simulink model "EKF_MODEL_needfix"  (R2023b)
settings: Solver=ode23tb  StartTime=0.0  StopTime=30  FixedStep=.001  RelTol=2e-1  EnableMultiTasking=on
StartFcn:
  | %tic
StopFcn:
  | %toc
model workspace (MAT data in the model file):
  DLCXref = [0 6.1 6.2 18 33 33.5 45 50 60]
  DLCXrefStanley = [0 1.2 2.4 3.6 4.8 6 7.2 8.4 9.44987166868 10.0991210544 10.1 10.1008789456 ... (38 elements, 1x38)]
  DLCYref = [0 0 -5 -3.875 -3.5 1 0 0 0]
  DLCYrefStanley = [0.1375 0.1375 0.1375 0.1375 0.1375 0.1375 0.1375 0.1375 -0.203439148031 -1.09615705337 -2.2 -3.30384294663 ... (38 elements, 1x38)]
  Downshift_Speeds = [9.5625 12.9375 16.3125 19.6875 23.0625 26.4375 29.8125 33.1875 36.5625 39.9375 43.3125 46.6875 ... (28 elements, 4x7)]
  EngRevLim = 7000
  Pedal_Positions = [0.1 0.4 0.5 0.9]
  Ts = 0.01
  Upshift_Speeds = [12.9375 16.3125 19.6875 33 26.4375 29.8125 33.1875 52.5 39.9375 43.3125 46.6875 77.25 ... (28 elements, 4x7)]
  VEH : object (value not decoded)
  a = 1.515
  b = 1.504
  for_ekf : mamfis (value not decoded)
  rayDirections = [0 0 0 0 0 0 0 0 0 0 0 0 ... (363 elements, 121x3)]
  rayLengths = [20 20 20 20 20 20 20 20 20 20 20 20 ... (121 elements, 121x1)]
  rayOrigins = [0.5 0.4 0.3 0.2 0.1 0 -0.1 -0.2 -0.3 -0.4 -0.5 0.5 ... (363 elements, 121x3)]
  theta = 1
  wf = 0.75
  wr = 1.25
symbols that are objects in the model workspace (value not decoded): VEH
undefined symbols (not defined in the file): DiscIntNeverNeededParam
libraries: simulink x14, autolibutils x7, slpidlib x2, vehdynlibdriver x2, vehdynlibviscommon x2, sim3dgroundtruthsensorlib x2, autolibtranscontrolscommon x1, autolibshared x1, sharedtransform x1, sharedTrackingLibrary x1, vehdynlibscenariocommon x1, vehdynlibsens x1
(part 2 of 4)

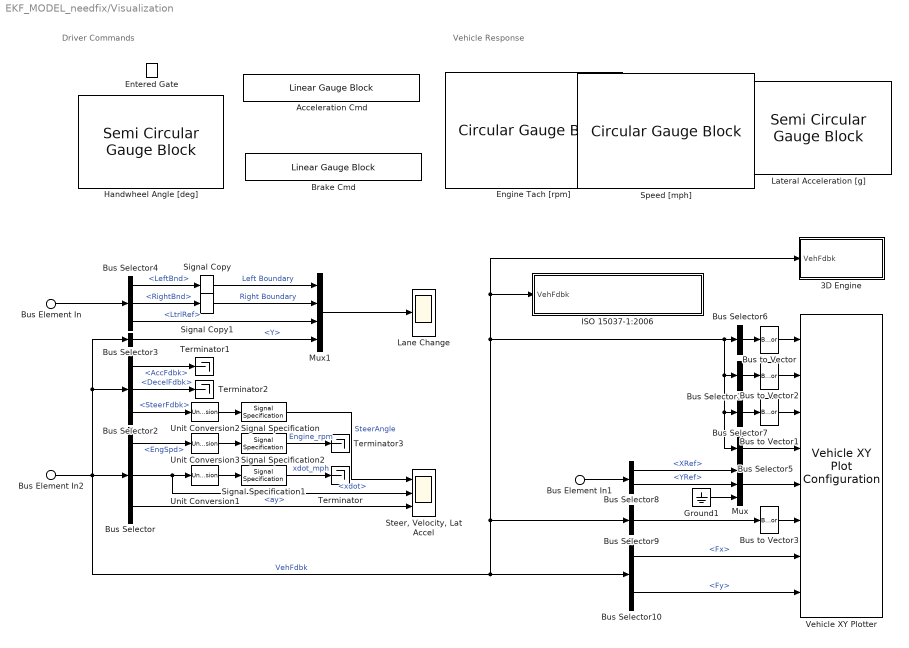
== system EKF_MODEL_needfix/Visualization ==
  note: Vehicle Response
  note: Driver Commands
  Bus Element In : Inport  PortName=Lane
  Bus Element In1 : Inport  PortName=Lane
  Bus Element In2 : Inport  Port=2  PortName=VehFdbk
  3D Engine : Subsystem  Variant=on  mask(3D Engine){engine3D=Disabled, use3DOp=off, SceneDesc=Double lane change, dt3D=.03, defaultPos=Recommended for scene, X_o=0, Y_o=5.7, Z_o=0, phi_o=0, theta_o=0, psi_o=0}
      mask prompts: engine3D "vdynblks:vehdynRefApp3DEng:blkPrm_engine3D"; use3DOp "Use default operating point"; SceneDesc "shared_sim3dblks:sim3dblkConfig:SceneDesc"; dt3D "vdynblks:vehdynRefApp3DEng:blkPrm_dt3D"; X_o "vdynblks:vehdynRefApp3DEng:blkPrm_X_o"; Y_o "vdynblks:vehdynRefApp3DEng:blkPrm_Y_o"; Z_o "vdynblks:vehdynRefApp3DEng:blkPrm_Z_o"; phi_o "vdynblks:vehdynRefApp3DEng:blkPrm_phi_o"; theta_o "vdynblks:vehdynRefApp3DEng:blkPrm_theta_o"; psi_o "vdynblks:vehdynRefApp3DEng:blkPrm_psi_o"
      mask help: This subsystem contains the interface blocks which permit the display of the vehicle in the 3D virtual environment. Enable it to view the simulation progress, disable it to inhibit the display.
      mask init:
      | GrndFdbkPath = find_system(bdroot(gcb), 'MatchFilter', @Simulink.match.allVariants,'BlockType','SubSystem','Name','Ground Feedback');
      | ManBlkName = 'Lane Change Reference Generator';
      | ManBlkPath = find_system(bdroot(gcb), 'MatchFilter', @Simulink.match.allVariants,'BlockType','SubSystem','Name',ManBlkName);
      | OpVarName = 'dlcSS35mph';
      | switch get_param(gcb,'engine3D')    
      |     case 'Disabled'
      |         try
      |             set_param(GrndFdbkPath{:},'OverrideUsingVariant','0');
      |         catch
      |             disp('Warning: Ground feedback source subsystem was not found. Ground feedback source remains unchanged.')
      |         end
      |         try
      |             if strcmp(get_param(gcb,'use3DOp'),'on') && strcmp(get_param(ManBlkPath{:},'ssMode'),'Resume from a workspace variable')
      |                 set_param(ManBlkPath{:},'ssVar',OpVarName);
      |             end
      |         catch
      |              disp('Warning: Maneuver source block not found. Steady state operating point not set')
      |         end
      |     case 'Enabled'
      |         try
      |             set_param(GrndFdbkPath{:},'OverrideUsingVariant','1');            
      |         catch
      |             disp('Warning: Ground feedback source subsystem was not found. Ground feedback source remains unchanged.')
      |         end
      |         try
      |             if strcmp(get_param(gcb,'use3DOp'),'on') && strcmp(get_param(ManBlkPath{:},'ssMode'),'Resume from a workspace variable')
      |                 set_param(ManBlkPath{:},'ssVar',[OpVarName '3D']);
      |             end
      |         catch
      |              disp('Warning: Maneuver source block not found. Steady state operating point not set')
      |         end
      |     otherwise
      | end
      settings: AttributesFormatString=|
      | %<SceneDesc>
      | %<engine3D>
      mask Help: eval('vdynblkshelp(''vdynblks3dengine'')');
      mask TypeOptions engine3D: vdynblks:vehdynRefApp3DEng:blkRdBt_engine3D_c1 | vdynblks:vehdynRefApp3DEng:blkRdBt_engine3D_c2
      mask Callback engine3D:
      | ManBlkName = 'Lane Change Reference Generator';
      | ManBlkPath = find_system(bdroot(gcb),'MatchFilter', @Simulink.match.allVariants,'BlockType','SubSystem','Name',ManBlkName);
      | switch get_param(gcb,'engine3D')
      |     case 'Disabled'
      |         try
      |             set_param(ManBlkPath{:},'use3DCones','off');
      |         catch
      |             disp('Warning: Lane change generator block not found in model')
      |         end
      |     case 'Enabled'
      |         try
      |             set_param(ManBlkPath{:},'use3DCones','on');
      |         catch
      |             disp('Warning: Lane change generator block not found in model')
      |         end
      |     otherwise
      | end
      mask TypeOptions SceneDesc: 3D Engine/Simulation 3D Scene Configuration/SceneDesc
      mask Callback SceneDesc:
      | defaultStatus = get_param(gcb,'defaultPos');
      | if strcmp(defaultStatus,'Recommended for scene')
      | sceneType = get_param(gcb,'SceneDesc');
      | switch sceneType
      |     case 'Straight road'
      |         set_param(gcb,'X_o', '-118')
      |         set_param(gcb,'Y_o', '5.7')
      |         set_param(gcb,'Z_o', '0')
      |         set_param(gcb,'phi_o', '0')
      |         set_param(gcb,'theta_o', '0')
      |         set_param(gcb,'psi_o', '0')
      |     case 'Curved road'
      |         set_param(gcb,'X_o', '0.2')
      |         set_param(gcb,'Y_o', '-1605.0')
      |         set_param(gcb,'Z_o', '0')
      |         set_param(gcb,'phi_o', '0')
      |         set_param(gcb,'theta_o', '0')
      |         set_param(gcb,'psi_o', '-156*pi/180')
      |     case 'Parking lot'
      |         set_param(gcb,'X_o', '-104.0')
      |         set_param(gcb,'Y_o', '-9.7')
      |         set_param(gcb,'Z_o', '0')
      |         set_param(gcb,'phi_o', '0')
      |         set_param(gcb,'theta_o', '0')
      |         set_param(gcb,'psi_o', '0')
      |     case 'Double lane change'
      |         set_param(gcb,'X_o', '0')
      |         set_param(gcb,'Y_o', '5.7')
      |         set_param(gcb,'Z_o', '0')
      |         set_param(gcb,'phi_o', '0')
      |         set_param(gcb,'theta_o', '0')
      |         set_param(gcb,'psi_o', '0')
      |     case 'Open surface'
      |         set_param(gcb,'X_o', '0')
      |         set_param(gcb,'Y_o', '0')
      |         set_param(gcb,'Z_o', '0')
      |         set_param(gcb,'phi_o', '0')
      |         set_param(gcb,'theta_o', '0')
      |         set_param(gcb,'psi_o', '0')
      |     case 'US highway'
      |         set_param(gcb,'X_o', '3592.00')
      |         set_param(gcb,'Y_o', '2617.00')
      |         set_param(gcb,'Z_o', '-1.0')
      |         set_param(gcb,'phi_o', '0')
      |         set_param(gcb,'theta_o', '0')
      |         set_param(gcb,'psi_o', '0')
      |     case 'US city block'
      |         set_param(gcb,'X_o', '-125.19')
      |         set_param(gcb,'Y_o', '1.65')
      |         set_param(gcb,'Z_o', '-0.04')
      |         set_param(gcb,'phi_o', '0')
      |         set_param(gcb,'theta_o', '0')
      |         set_param(gcb,'psi_o', '0')
      |     case 'Large parking lot'
      |         set_param(gcb,'X_o', '45.0')
      |         set_param(gcb,'Y_o', '54.7')
      |         set_param(gcb,'Z_o', '0.0')
      |         set_param(gcb,'phi_o', '0')
      |         set_param(gcb,'theta_o', '0')
      |         set_param(gcb,'psi_o', '-pi/2')
      |     case 'Virtual Mcity'
      |         set_param(gcb,'X_o', '-26.0')
      |         set_param(gcb,'Y_o', '76.0')
      |         set_param(gcb,'Z_o', '0.0')
      |         set_param(gcb,'phi_o', '0')
      |         set_param(gcb,'theta_o', '0')
      |         set_param(gcb,'psi_o', '-40*pi/180')
      |    case 'Suburban'
      |         set_param(gcb,'X_o', '60')
      |         set_param(gcb,'Y_o', '-41.7')
      |         set_param(gcb,'Z_o', '0.0')
      |         set_param(gcb,'phi_o', '0')
      |         set_param(gcb,'theta_o', '0')
      |         set_param(gcb,'psi_o', '-0.192')
      |     otherwise
      |         set_param(gcb,'X_o', '0')
      |         set_param(gcb,'Y_o', '0')
      |         set_param(gcb,'Z_o', '0')
      |         set_param(gcb,'phi_o', '0')
      |         set_param(gcb,'theta_o', '0')
      |         set_param(gcb,'psi_o', '0')
      | end
      | end
      mask TypeOptions defaultPos: vdynblks:vehdynRefApp3DEng:blkRdBt_defaultPos_c1 | vdynblks:vehdynRefApp3DEng:blkRdBt_defaultPos_c2
      mask DialogControl engineConfig Prompt: vdynblks:vehdynRefApp3DEng:blkDlg_engineConfig
      mask DialogControl engine3D Prompt: 3D Engine
      mask DialogControl SceneDesc Prompt: Scene name:
      mask DialogControl dt3D Prompt: 3D Engine frame rate, dt3D [s]:
      mask DialogControl posSetup Prompt: vdynblks:vehdynRefApp3DEng:blkDlg_posSetup
      mask DialogControl posSetupDesc Prompt: vdynblks:vehdynRefApp3DEng:blkDisTxt_posSetupDesc
      mask DialogControl X_o Prompt: Initial longitudinal position, X_o [m]:
      mask DialogControl Y_o Prompt: Initial lateral position, Y_o [m]:
      mask DialogControl Z_o Prompt: Initial vertical position, Z_o [m]:
      mask DialogControl phi_o Prompt: Initial roll angle, phi_o [rad]:
      mask DialogControl theta_o Prompt: Initial pitch angle, theta_o [rad]:
      mask DialogControl psi_o Prompt: Initial yaw angle, psi_o [rad]:
      mask DialogControl setModelPos Prompt: vdynblks:vehdynRefApp3DEng:blkDlg_setModelPos
      mask DialogControl setModelPos Callback:
      | if strcmp(get_param(bdroot(gcb),'SimulationStatus'),'stopped')
      |     sceneType = get_param(gcb,'SceneDesc');
      |     rootModel = bdroot(gcb);
      |     ws = get_param(rootModel, 'modelworkspace');
      |     VEH = getVariable(ws,'VEH');
      |     ParamList={'X_o',[1,1],{};'Y_o',[1,1],{};'Z_o',[1,1],{};'phi_o',[1,1],{'gte',-pi/2;'lte',pi/2};'theta_o',[1,1],{'gte',-pi/2;'lte',pi/2};'psi_o',[1,1],{'gte',-2*pi;'lte',2*pi}};
      |     paramStruct = autoblkscheckparams(gcb, '3D Engine',ParamList);
      |     VEH.InitialLongPosition = paramStruct.X_o;
      |     VEH.InitialLatPosition = paramStruct.Y_o;
      |     VEH.InitialVertPosition = paramStruct.Z_o;
      |     VEH.InitialRollAngle = paramStruct.phi_o;
      |     VEH.InitialPitchAngle = paramStruct.theta_o;
      |     VEH.InitialYawAngle = paramStruct.psi_o;
      |     assignin(ws,'VEH',VEH);
      |     modelList = {'PassVeh14DOF','PassVeh7DOF'};
      |     for idx =1:length(modelList)
      | %         try
      |             load_system(modelList{idx});
      |             ws = get_param(modelList{idx}, 'modelworkspace');
      |             assignin(ws,'VEH',VEH);
      |             save_system(modelList{idx});
      |             close_system(modelList{idx});
      | %         catch
      | %             disp(['Cannot find ' modelList{idx}])
      | %         end
      |     end
      | end
      mask Display: disp('3D Engine')
  Acceleration Cmd : LinearGaugeBlock  LabelPosition=Hide  ScaleMax=1  TickInterval=0.20000000000000001
  Brake Cmd : LinearGaugeBlock  LabelPosition=Hide  ScaleMax=1  TickInterval=0.20000000000000001
  Bus Selector : BusSelector  OutputSignals=Driveline.EngSpd,Body.BdyFrm.Cg.Vel.xdot,Body.BdyFrm.Cg.Acc.ay
  Bus Selector1 : BusSelector  OutputSignals=Body.InertFrm.Cg.Ang.phi,Body.InertFrm.Cg.Ang.theta,Body.InertFrm.Cg.Ang.psi  OutputAsBus=on
  Bus Selector10 : BusSelector  OutputSignals=Wheels.TireFrame.Fx,Wheels.TireFrame.Fy
  Bus Selector2 : BusSelector  OutputSignals=Driver.AccFdbk,Driver.DecelFdbk,Driver.SteerFdbk
  Bus Selector3 : BusSelector  OutputSignals=Body.InertFrm.Cg.Disp.Y
  Bus Selector4 : BusSelector  OutputSignals=LeftBnd,RightBnd,LtrlRef
  Bus Selector5 : BusSelector  OutputSignals=Driveline.WhlAng  OutputAsBus=on
  Bus Selector6 : BusSelector  OutputSignals=Body.InertFrm.Geom.Disp.X,Body.InertFrm.Geom.Disp.Y,Body.InertFrm.Geom.Disp.Z  OutputAsBus=on
  Bus Selector7 : BusSelector  OutputSignals=Body.InertFrm.Geom.Vel.Xdot,Body.InertFrm.Geom.Vel.Ydot,Body.InertFrm.Geom.Vel.Zdot  OutputAsBus=on
  Bus Selector8 : BusSelector  OutputSignals=XRef,YRef
  Bus Selector9 : BusSelector  OutputSignals=Driveline.EngSpd,Driveline.Gear  OutputAsBus=on
  Bus to Vector{,1..3} (4 alike) : BusToVector
  Engine Tach [rpm] : CircularGaugeBlock  LabelPosition=Hide  ScaleMax=8000  TickInterval=1000
  Entered Gate : LampBlock  LabelPosition=Hide
  Ground1 : Ground
  Handwheel Angle [deg] : SemiCircularGaugeBlock  LabelPosition=Hide  ScaleMin=-300  ScaleMax=300  TickInterval=60
  ISO 15037-1:2006 : Subsystem  StopFcn=|  Variant=on  VariantControlMode=label  LabelModeActiveChoice=0  mask(ISO 15037-1:2006){Measurement=Disabled}
      | switch get_param(gcb,'Measurement')
      |     case 'Enabled'
      |        p=slproject.getCurrentProject;
      |        projectRoot=p.RootFolder;
      |        SySFolder=fullfile(projectRoot, 'System');
      |        Simulink.sdi.loadView([SySFolder filesep 'ISO15037_1_2006E.mldatx']);
      |        Simulink.sdi.view;
      | end
      mask prompts: Measurement "ISO Measurements"
      mask help: Enables display of ISO 15037-1:2006 standard measurement signals in the Simulation Data Inspector.
      mask init:
      | switch get_param(gcb,'Measurement')
      |     case 'Disabled'
      |         set_param(gcb,'OverrideUsingVariant','0')
      |     case 'Enabled'
      |        set_param(gcb,'OverrideUsingVariant','1')
      |     otherwise
      |        set_param(gcb,'OverrideUsingVariant','0')
      | end
      settings: AttributesFormatString=%<Measurement>
      mask Help: eval('vdynblkshelp(''iso15037'')');
      mask TypeOptions Measurement: Enabled | Disabled
      mask Callback Measurement:
      | switch get_param(gcb,'Measurement')
      |     case 'Disabled'
      |         set_param(gcb,'OverrideUsingVariant','0')
      |     case 'Enabled'
      |        set_param(gcb,'OverrideUsingVariant','1')
      |     otherwise
      |        set_param(gcb,'OverrideUsingVariant','0')
      | end
      mask Display: disp('ISO 15037-1:2006')
  Lane Change : Scope
  Lateral Acceleration [g] : SemiCircularGaugeBlock  LabelPosition=Hide  ScaleMin=-1  ScaleMax=1  TickInterval=0.5
  Mux : Mux  Inputs=3
  Mux1 : Mux
  Signal Copy : SignalConversion  OverrideOpt=off
  Signal Copy1 : SignalConversion  OverrideOpt=off
  Signal Specification : SignalSpecification  Unit=deg
  Signal Specification1 : SignalSpecification  Unit=mph
  Signal Specification2 : SignalSpecification  Unit=rpm
  Speed [mph] : CircularGaugeBlock  LabelPosition=Hide  TickInterval=10
  "Steer, Velocity, Lat Accel" : Scope  NumInputPorts=3
  Terminator{,1..3} (4 alike) : Terminator
  Unit Conversion1 : UnitConversion
  Unit Conversion2 : UnitConversion
  Unit Conversion3 : UnitConversion
  Vehicle XY Plotter : vehdynlibviscommon/Vehicle XY Plot Configuration  extRef=on  extStats=on  extTireF=on  a=VEH.FrontAxlePositionfromCG  b=VEH.RearAxlePositionfromCG  w=VEH.TrackWidth  figBorder=10  bufferSize=1024  velNorm=5  tireFNorm=1000  pltDT=.1
  wires:
  Signal Specification/1 -> "Steer, Velocity, Lat Accel"/1  "SteerAngle"
  Bus Selector/3 -> "Steer, Velocity, Lat Accel"/3  "<ay>"
  Bus Selector/2 -> "Steer, Velocity, Lat Accel"/2, Unit Conversion1/1  "<xdot>"
  Unit Conversion2/1 -> Signal Specification/1
  Unit Conversion1/1 -> Signal Specification1/1
  Signal Specification1/1 -> Terminator/1  "xdot_mph"
  Bus Selector4/2 -> Signal Copy1/1  "<RightBnd>"
  Mux1/1 -> Lane Change/1
  Bus Selector3/1 -> Mux1/4  "<Y>"
  Bus Selector4/1 -> Signal Copy/1  "<LeftBnd>"
  Bus Selector4/3 -> Mux1/3  "<LtrlRef>"
  Bus Selector2/3 -> Unit Conversion2/1  "<SteerFdbk>"
  Bus Selector2/1 -> Terminator1/1  "<AccFdbk>"
  Bus Selector2/2 -> Terminator2/1  "<DecelFdbk>"
  Signal Specification2/1 -> Terminator3/1  "Engine_rpm"
  Unit Conversion3/1 -> Signal Specification2/1
  Bus Selector/1 -> Unit Conversion3/1  "<EngSpd>"
  Bus Selector7/1 -> Bus to Vector1/1
  Bus to Vector/1 -> Vehicle XY Plotter/1
  Bus Selector6/1 -> Bus to Vector/1
  Bus to Vector1/1 -> Vehicle XY Plotter/3
  Bus Selector1/1 -> Bus to Vector2/1
  Bus Element In2/1 -> Bus Selector3/1, Bus Selector2/1, ISO 15037-1:2006/1(VehFdbk), 3D Engine/1(VehFdbk), Bus Selector5/1, Bus Selector7/1, Bus Selector1/1, Bus Selector6/1, Bus Selector9/1, Bus Selector10/1, Bus Selector/1  "VehFdbk"
  Mux/1 -> Vehicle XY Plotter/5
  Ground1/1 -> Mux/3
  Bus Selector8/1 -> Mux/1  "<XRef>"
  Bus Element In/1 -> Bus Selector4/1
  Bus Selector8/2 -> Mux/2  "<YRef>"
  Bus to Vector3/1 -> Vehicle XY Plotter/6
  Bus Selector9/1 -> Bus to Vector3/1
  Bus to Vector2/1 -> Vehicle XY Plotter/2
  Bus Selector5/1 -> Vehicle XY Plotter/4
  Bus Selector10/2 -> Vehicle XY Plotter/8  "<Fy>"
  Bus Selector10/1 -> Vehicle XY Plotter/7  "<Fx>"
  Signal Copy/1 -> Mux1/1  "Left Boundary"
  Signal Copy1/1 -> Mux1/2  "Right Boundary"
  Bus Element In1/1 -> Bus Selector8/1

== system EKF_MODEL_needfix/imu ==
  In1 : Inport
  Demux1 : Demux  Outputs=6
  Mux2 : Mux  Inputs=3
  Out4 : Outport
  wires:
  Demux1/2 -> Mux2/2
  Demux1/1 -> Mux2/1
  Demux1/6 -> Mux2/3
  In1/1 -> Demux1/1
  Mux2/1 -> Out4/1

== system EKF_MODEL_needfix/imu signal ==
  xdot : Inport
  Add1 : Sum
  Constant2 : Constant  Value=0.06
  MATLAB Function1 : MATLAB Function  TreatAsAtomicUnit=on
  Zero-Order Hold5 : ZeroOrderHold  SampleTime=0.01
  u : Outport
  wires:
  MATLAB Function1/1(randomMatrix) -> Add1/1
  Zero-Order Hold5/1 -> u/1
  Constant2/1 -> MATLAB Function1/1(variance)
  Add1/1 -> Zero-Order Hold5/1
  xdot/1 -> Add1/2

== system EKF_MODEL_needfix/model data ==
  In1 : Inport
  In2 : Inport  Port=2
  Inport : Inport  Port=3
  Subsystem : Subsystem
  <body_a> : Outport
  <imu> : Outport  Port=2
  <steerangle> : Outport  Port=3
  <wheelspeed> : Outport  Port=4
  <EngTrq> : Outport  Port=5
  <xdot> : Outport  Port=6
  <ydot> : Outport  Port=7
  <r> : Outport  Port=8
  wires:
  Subsystem/1(<body_a>) -> <body_a>/1
  Subsystem/2(<imu>) -> <imu>/1
  Subsystem/5(<xdot>) -> <xdot>/1
  Subsystem/3(<steerangle>) -> <steerangle>/1
  Subsystem/7(<r>) -> <r>/1
  Subsystem/6(<ydot>) -> <ydot>/1
  Subsystem/4(<EngTrq>) -> <EngTrq>/1
  Inport/1 -> <wheelspeed>/1
  In2/1 -> Subsystem/2(In2)
  In1/1 -> Subsystem/1(In1)

== system EKF_MODEL_needfix/wheel speed adjust ==
  <wheelspeed> : Inport
  Demux : Demux
  Mux1 : Mux
  wheel_speed : Outport
  wires:
  Demux/4 -> Mux1/3
  <wheelspeed>/1 -> Demux/1
  Demux/2 -> Mux1/1
  Demux/1 -> Mux1/2
  Mux1/1 -> wheel_speed/1
  Demux/3 -> Mux1/4

== system EKF_MODEL_needfix/wheel speed signal ==
  y_ideal : Inport
  moise : Inport  Port=2
  Add : Sum
  Constant1 : Constant  Value=0.303
  Product : Product
  Zero-Order Hold1 : ZeroOrderHold  SampleTime=0.01
  y_real : Outport
  wires:
  Zero-Order Hold1/1 -> y_real/1
  Add/1 -> Zero-Order Hold1/1
  moise/1 -> Add/2
  Product/1 -> Add/1
  Constant1/1 -> Product/2
  y_ideal/1 -> Product/1

== system EKF_MODEL_needfix/Controllers/Active Differential Control ==
  note: 1) Add Subsystem or Model blocks as valid variant choices.
      | 2) You cannot connect blocks at this level. At simulation, connectivity is automatically
      | determined, based on the active variant and port name matching.
  Accel : Inport
  BrkCmd : Inport  Port=2
  Steer : Inport  Port=3
  GearFdbk : Inport  Port=4
  Omega : Inport  Port=5  Unit=rad/s
  axayaz : Inport  Port=6
  pqr : Inport  Port=7
  No Control : Subsystem  VariantControl=0
  Rear Diff Controller : Subsystem  TreatAsAtomicUnit=on  SystemSampleTime=.01  VariantControl=1
  DiffPrsCmd : Outport  VectorParamsAs1DForOutWhenUnconnected=off
  TrqCmd : Outport  Port=2  VectorParamsAs1DForOutWhenUnconnected=off

== system EKF_MODEL_needfix/Controllers/Brake Pressure Control ==
  note: 1) Add Subsystem or Model blocks as valid variant choices.
      | 2) You cannot connect blocks at this level. At simulation, connectivity is automatically
      | determined, based on the active variant and port name matching.
  DecelFdbk : Inport
  Omega : Inport  Port=2
  Accel : Inport  Port=3
  AccelFdbk : Inport  Port=4
  BrkPrs : Inport  Port=5
  Bang Bang ABS : Subsystem  VariantControl=1
  Five-State ABS and TCS : Subsystem  VariantControl=2
  Open Loop : Subsystem  VariantControl=0
  ABSFlag : Outport  VectorParamsAs1DForOutWhenUnconnected=off
  BrkPrsCmd : Outport  Port=2  VectorParamsAs1DForOutWhenUnconnected=off
  TCSFlag : Outport  Port=3  VectorParamsAs1DForOutWhenUnconnected=off

== system EKF_MODEL_needfix/Controllers/ECU ==
  DiffTrqCmd : Inport
  <Accel> : Inport  Port=2
  EngSpd : Inport  Port=3
  ABSFlag : Inport  Port=4
  First Order Hold : FirstOrderHold  ErrorTolerance=100
  Torque Cmd : Subsystem  TreatAsAtomicUnit=on  SystemSampleTime=.01
  EngTrqCmd : Outport  VectorParamsAs1DForOutWhenUnconnected=off
  wires:
  First Order Hold/1 -> EngTrqCmd/1
  DiffTrqCmd/1 -> Torque Cmd/1(DiffTrqCmd)
  <Accel>/1 -> Torque Cmd/2(<Accel>)
  EngSpd/1 -> Torque Cmd/3(EngSpd)
  Torque Cmd/1(EngTrqCmd) -> First Order Hold/1
  ABSFlag/1 -> Torque Cmd/4(ABSFlag)

== system EKF_MODEL_needfix/Controllers/Transmission Controller ==
  Accel : Inport
  BrkCmd : Inport  Port=2
  GearReq : Inport  Port=3
  EngSpd : Inport  Port=4
  Omega : Inport  Port=5  Unit=rad/s
  ABSFlag : Inport  Port=6
  UpReq : Inport  Port=7
  DownReq : Inport  Port=8  Unit=rad/s
  Driver - No Clutch : Subsystem  VariantControl=1
  PRNDL Controller : Subsystem  VariantControl=3
  Paddles : Subsystem  VariantControl=2
  Transmission Controller : Subsystem  VariantControl=0
  " Gear" : Outport  VectorParamsAs1DForOutWhenUnconnected=off

== system EKF_MODEL_needfix/Driver Commands/Driver Commands ==
  VehRef : Inport
  VehFdbk : Inport  Port=2
  SteerCmd : Inport  Port=3
  Accel : Inport  Port=4
  Brake : Inport  Port=5
  Gear : Inport  Port=6
  Longitudinal Driver : Subsystem  VariantControl=driverType==1
  Open Loop : Subsystem  VariantControl=driverType==4
  Predictive Driver : Subsystem  VariantControl=driverType==2
  Predictive Stanley Driver : Subsystem  VariantControl=driverType==3
  " Driver" : Outport  VectorParamsAs1DForOutWhenUnconnected=off

== system EKF_MODEL_needfix/Environment/Ground Feedback ==
  Friction : Inport
  VehFdbk : Inport  Port=2
  3D Engine : Subsystem  VariantControl=1
  Constant : Subsystem  VariantControl=0
  Ground : Outport  VectorParamsAs1DForOutWhenUnconnected=off

== system EKF_MODEL_needfix/Passenger Vehicle/Body, Suspension, Wheels ==
  note: 1) Add additional chassis Model reference blocks as valid variant choices for your specific use cases.
      | 2) You cannot connect blocks at this level. At simulation, connectivity is automatically
      | determined, based on the active variant and port name matching.
  WindXYZ : Inport
  Ground : Inport  Port=2  PortDimensions=4
  DCM : Inport  Port=3
  Friction : Inport  Port=4  PortDimensions=4
  WhlAng : Inport  Port=5
  AxlTrq : Inport  Port=6
  BrkPrs : Inport  Port=7
  PassVeh14DOF : ModelReference  DisableCoverage=on  ModelNameDialog=PassVeh14DOF  VariantControl=3  ModelReferenceVersion=6.11
  PassVeh7DOF : ModelReference  ModelNameDialog=PassVeh7DOF  SimulationMode=Normal  VariantControl=1  ModelReferenceVersion=6.2
  Veh : Outport  VectorParamsAs1DForOutWhenUnconnected=off
  Wheels : Outport  Port=2  VectorParamsAs1DForOutWhenUnconnected=off

== system EKF_MODEL_needfix/Passenger Vehicle/Chassis Input ==
  Env : Inport
  Driveline : Inport  Port=2
  Bus Selector1 : BusSelector  OutputSignals=Gnd.z.G_FL_z,Gnd.z.G_FR_z,Gnd.z.G_RL_z,Gnd.z.G_RR_z
  Bus Selector2 : BusSelector  OutputSignals=Wind
  Bus Selector3 : BusSelector  OutputSignals=Gnd.mu.mu_FL,Gnd.mu.mu_FR,Gnd.mu.mu_RL,Gnd.mu.mu_RR
  Bus Selector4 : BusSelector  OutputSignals=WhlAng,AxlTrq,BrkPrs
  Bus Selector5 : BusSelector  OutputSignals=Gnd.DCM
  Vector Concatenate : Concatenate  NumInputs=4
  Vector Concatenate1 : Concatenate  NumInputs=4
  Wind : Outport  VectorParamsAs1DForOutWhenUnconnected=off
  Gnd : Outport  Port=2  VectorParamsAs1DForOutWhenUnconnected=off
  DCM : Outport  Port=3  VectorParamsAs1DForOutWhenUnconnected=off
  mu : Outport  Port=4  VectorParamsAs1DForOutWhenUnconnected=off
  WhlAng : Outport  Port=5  VectorParamsAs1DForOutWhenUnconnected=off
  AxlTrq : Outport  Port=6  VectorParamsAs1DForOutWhenUnconnected=off
  BrkPrs : Outport  Port=7  VectorParamsAs1DForOutWhenUnconnected=off
  wires:
  Env/1 -> Bus Selector5/1, Bus Selector3/1, Bus Selector1/1, Bus Selector2/1
  Bus Selector2/1 -> Wind/1  "<Wind>"
  Bus Selector3/1 -> Vector Concatenate/1  "<mu_FL>"
  Bus Selector3/2 -> Vector Concatenate/2  "<mu_FR>"
  Bus Selector3/3 -> Vector Concatenate/3  "<mu_RL>"
  Bus Selector3/4 -> Vector Concatenate/4  "<mu_RR>"
  Vector Concatenate/1 -> mu/1
  Bus Selector1/1 -> Vector Concatenate1/1  "<G_FL_z>"
  Bus Selector1/2 -> Vector Concatenate1/2  "<G_FR_z>"
  Bus Selector1/3 -> Vector Concatenate1/3  "<G_RL_z>"
  Bus Selector1/4 -> Vector Concatenate1/4  "<G_RR_z>"
  Vector Concatenate1/1 -> Gnd/1
  Driveline/1 -> Bus Selector4/1
  Bus Selector4/2 -> AxlTrq/1  "<AxlTrq>"
  Bus Selector4/1 -> WhlAng/1  "<WhlAng>"
  Bus Selector4/3 -> BrkPrs/1  "<BrkPrs>"
  Bus Selector5/1 -> DCM/1  "<DCM>"

== system EKF_MODEL_needfix/Passenger Vehicle/Chassis Output ==
  Veh : Inport
  Wheels : Inport  Port=2
  Out Bus Element4 : Outport  PortName=VehFdbk
  Out Bus Element1 : Outport  Port=2  PortName=WheelsFdbk
  wires:
  Veh/1 -> Out Bus Element4/1
  Wheels/1 -> Out Bus Element1/1

== system EKF_MODEL_needfix/Passenger Vehicle/Driveline Input ==
  Cntrl : Inport
  Driver : Inport  Port=2
  EngTrqCmd : Inport  Port=3
  Wheels : Inport  Port=4
  Bus Selector1 : BusSelector  OutputSignals=SteerCmd
  Bus Selector2 : BusSelector  OutputSignals=TireFrame.Omega
  Bus Selector3 : BusSelector  OutputSignals=Transmission.GearCmd,Brake.BrkPrsCmd,Diff.DiffPrsCmd
  Bus Selector4 : BusSelector  OutputSignals=EngTrq
  Data Type Conversion : DataTypeConversion  SaturateOnIntegerOverflow=off  RndMeth=Floor
  Steer : Outport  VectorParamsAs1DForOutWhenUnconnected=off
  EngTrq : Outport  Port=2  VectorParamsAs1DForOutWhenUnconnected=off
  GearCmd : Outport  Port=3  VectorParamsAs1DForOutWhenUnconnected=off
  BrkPrsCmd : Outport  Port=4  VectorParamsAs1DForOutWhenUnconnected=off
  Omega : Outport  Port=5  VectorParamsAs1DForOutWhenUnconnected=off
  DiffPrsCmd : Outport  Port=6  VectorParamsAs1DForOutWhenUnconnected=off
  wires:
  Cntrl/1 -> Bus Selector3/1
  Bus Selector3/1 -> Data Type Conversion/1  "<GearCmd>"
  Driver/1 -> Bus Selector1/1
  Wheels/1 -> Bus Selector2/1
  Bus Selector2/1 -> Omega/1  "<Omega>"
  Bus Selector3/2 -> BrkPrsCmd/1  "<BrkPrsCmd>"
  EngTrqCmd/1 -> Bus Selector4/1
  Bus Selector1/1 -> Steer/1  "<SteerCmd>"
  Bus Selector4/1 -> EngTrq/1  "<EngTrq>"
  Bus Selector3/3 -> DiffPrsCmd/1  "<DiffPrsCmd>"
  Data Type Conversion/1 -> GearCmd/1

== system EKF_MODEL_needfix/Passenger Vehicle/Driveline Output ==
  WhlAng : Inport
  AxlTrq : Inport  Port=2
  BrkPrs : Inport  Port=3
  EngSpd : Inport  Port=4
  PropShftSpd : Inport  Port=5
  StrWhlTrq : Inport  Port=6
  Gear : Inport  Port=7
  Bus Creator1 : BusCreator  Inputs=6
  Bus Creator2 : BusCreator  Inputs=1
  Driveline : Outport  VectorParamsAs1DForOutWhenUnconnected=off
  Steering : Outport  Port=2  VectorParamsAs1DForOutWhenUnconnected=off
  wires:
  Bus Creator1/1 -> Driveline/1  "Driveline"
  PropShftSpd/1 -> Bus Creator1/5  "PropShftSpd"
  AxlTrq/1 -> Bus Creator1/2  "AxlTrq"
  WhlAng/1 -> Bus Creator1/1  "WhlAng"
  EngSpd/1 -> Bus Creator1/4  "EngSpd"
  BrkPrs/1 -> Bus Creator1/3  "BrkPrs"
  StrWhlTrq/1 -> Bus Creator2/1  "StrWhlTrq"
  Bus Creator2/1 -> Steering/1  "Steering"
  Gear/1 -> Bus Creator1/6  "Gear"

== system EKF_MODEL_needfix/Passenger Vehicle/Engine ==
  note: 1) Add additional Engine Model reference blocks as valid variant choices for your specific use cases.
      | 2) You cannot connect blocks at this level. At simulation, connectivity is automatically
      | determined, based on the active variant and port name matching.
  TrqCmd : Inport
  EngSpd : Inport  Port=2  Unit=rad/s
  Ideal Mapped Engine : ModelReference  DisableCoverage=on  ModelNameDialog=SiMappedEngineV  VariantControl=0  ModelReferenceVersion=6.0
  EngTrq : Outport  VectorParamsAs1DForOutWhenUnconnected=off

== system EKF_MODEL_needfix/Passenger Vehicle/Engine Input ==
  Cntrl : Inport
  Driveline : Inport  Port=2
  Bus Selector : BusSelector  OutputSignals=ECU.EngTrqCmd
  Bus Selector1 : BusSelector  OutputSignals=EngSpd
  EngTrqCmd : Outport  VectorParamsAs1DForOutWhenUnconnected=off
  EngSpd : Outport  Port=2  VectorParamsAs1DForOutWhenUnconnected=off
  wires:
  Driveline/1 -> Bus Selector1/1
  Cntrl/1 -> Bus Selector/1
  Bus Selector/1 -> EngTrqCmd/1  "<EngTrqCmd>"
  Bus Selector1/1 -> EngSpd/1  "<EngSpd>"

== system EKF_MODEL_needfix/Passenger Vehicle/Engine Output ==
  "EngTrq " : Inport
  Bus Creator : BusCreator  Inputs=1
  Eng : Outport  VectorParamsAs1DForOutWhenUnconnected=off
  wires:
  "EngTrq "/1 -> Bus Creator/1  "EngTrq"
  Bus Creator/1 -> Eng/1

== system EKF_MODEL_needfix/Passenger Vehicle/Pedal Cluster Input ==
  Driver : Inport
  Driveline : Inport  Port=2
  Steering : Inport  Port=3
  Bus Selector : BusSelector  OutputSignals=SteerCmd,AccelCmd,DecelCmd,GearCmd
  Bus Selector1 : BusSelector  OutputSignals=BrkPrs
  Bus Selector2 : BusSelector  OutputSignals=StrWhlTrq
  SteerCmd : Outport  VectorParamsAs1DForOutWhenUnconnected=off
  AccelCmd : Outport  Port=2  VectorParamsAs1DForOutWhenUnconnected=off
  DecelCmd : Outport  Port=3  VectorParamsAs1DForOutWhenUnconnected=off
  GearCmd : Outport  Port=4  VectorParamsAs1DForOutWhenUnconnected=off
  BrkPrs : Outport  Port=5  VectorParamsAs1DForOutWhenUnconnected=off
  StrWhlTrq : Outport  Port=6  VectorParamsAs1DForOutWhenUnconnected=off
  wires:
  Bus Selector/2 -> AccelCmd/1  "<AccelCmd>"
  Driver/1 -> Bus Selector/1
  Bus Selector/3 -> DecelCmd/1  "<DecelCmd>"
  Bus Selector/4 -> GearCmd/1  "<GearCmd>"
  Bus Selector/1 -> SteerCmd/1  "<SteerCmd>"
  Driveline/1 -> Bus Selector1/1
  Bus Selector1/1 -> BrkPrs/1  "<BrkPrs>"
  Steering/1 -> Bus Selector2/1
  Bus Selector2/1 -> StrWhlTrq/1  "<StrWhlTrq>"

== system EKF_MODEL_needfix/Passenger Vehicle/Pedal Cluster Output ==
  SteerFdbk : Inport
  AccFdbk : Inport  Port=2
  DecelFdbk : Inport  Port=3
  GearFdbk : Inport  Port=4
  Bus Creator1 : BusCreator  Inputs=4
  Signal Specification : SignalSpecification  Unit=rad
  Signal Specification1 : SignalSpecification  Unit=1
  Signal Specification2 : SignalSpecification  Unit=1
  Signal Specification3 : SignalSpecification  Unit=1
  OperatorFdbk : Outport
  wires:
  Signal Specification1/1 -> Bus Creator1/2  "AccFdbk"
  Signal Specification3/1 -> Bus Creator1/4  "GearFdbk"
  AccFdbk/1 -> Signal Specification1/1
  DecelFdbk/1 -> Signal Specification2/1
  GearFdbk/1 -> Signal Specification3/1
  Signal Specification/1 -> Bus Creator1/1  "SteerFdbk"
  SteerFdbk/1 -> Signal Specification/1
  Bus Creator1/1 -> OperatorFdbk/1
  Signal Specification2/1 -> Bus Creator1/3  "DecelFdbk"

== system EKF_MODEL_needfix/Passenger Vehicle/Pedal Cluster and Cabin ==
  note: Placeholder for introducing faults, detailed actuator behavior,
      | interactions of other systems with a human interface such
      | as changes in power steering and braking assistance.
  SteerCmd : Inport
  AccCmd : Inport  Port=2
  DecelCmd : Inport  Port=3
  GearCmd : Inport  Port=4
  BrkPrs : Inport  Port=5
  StrWhlTrq : Inport  Port=6
  Brake Pedal : Subsystem
  Dead Zone2 : DeadZone  LowerValue=0  UpperValue=.01  ZeroCross=off
  Dead Zone3 : DeadZone  LowerValue=-.01  UpperValue=.01  ZeroCross=off
  Terminator : Terminator
  Terminator1 : Terminator
  SteerFdbk : Outport
  AccFdbk : Outport  Port=2
  DecelFdbk : Outport  Port=3
  GearFdbk : Outport  Port=4
  wires:
  SteerCmd/1 -> Dead Zone3/1
  AccCmd/1 -> Dead Zone2/1
  DecelCmd/1 -> Brake Pedal/1(DecelCmd)
  GearCmd/1 -> GearFdbk/1
  BrkPrs/1 -> Terminator/1
  StrWhlTrq/1 -> Terminator1/1
  Brake Pedal/1(DecelFdbk) -> DecelFdbk/1
  Dead Zone2/1 -> AccFdbk/1
  Dead Zone3/1 -> SteerFdbk/1

== system EKF_MODEL_needfix/Passenger Vehicle/Steering, Transmission, Driveline and Brakes ==
  note: 1) Add additional Driveline Model reference blocks as valid variant choices for your specific use cases.
      | 2) You cannot connect blocks at this level. At simulation, connectivity is automatically
      | determined, based on the active variant and port name matching.
  SteerHWCmd : Inport
  EngTrq : Inport  Port=2
  GearCmd : Inport  Port=3  OutDataTypeStr=int8
  BrkPrsCmd : Inport  Port=4  PortDimensions=4
  Omega : Inport  Port=5
  DiffPrsCmd : Inport  Port=6
  Driveline Ideal Fixed Gear : ModelReference  DisableCoverage=on  ModelNameDialog=Driveline  VariantControl=0  ModelReferenceVersion=6.0
  WhlAng : Outport  VectorParamsAs1DForOutWhenUnconnected=off
  AxlTrq : Outport  Port=2  VectorParamsAs1DForOutWhenUnconnected=off
  BrkPrs : Outport  Port=3  PortDimensions=4  VectorParamsAs1DForOutWhenUnconnected=off
  EngSpd : Outport  Port=4  Unit=rad/s  VectorParamsAs1DForOutWhenUnconnected=off
  PropShftSpd : Outport  Port=5  VectorParamsAs1DForOutWhenUnconnected=off
  StrWhlTrq : Outport  Port=6  VectorParamsAs1DForOutWhenUnconnected=off
  Gear : Outport  Port=7  VectorParamsAs1DForOutWhenUnconnected=off

== system EKF_MODEL_needfix/Subsystem1/Subsystem2 ==
  In1 : Inport
  Add : Sum
  Constant : Constant
  Constant5 : Constant  Value=100
  Divide : Product  Inputs=*/
  variance : Outport
  wires:
  Add/1 -> Divide/1
  In1/1 -> Add/1
  Constant5/1 -> Divide/2
  Constant/1 -> Add/2
  Divide/1 -> variance/1

== system EKF_MODEL_needfix/Visualization/3D Engine ==
  note: 1) Add Subsystem or Model blocks as valid variant choices.
      | 2) You cannot connect blocks at this level. At simulation, connectivity is automatically
      | determined, based on the active variant and port name matching.
  VehFdbk : Inport
  3D Engine : Subsystem  VariantControl=engine3D==1
  3D Engine Disabled : Subsystem  VariantControl=engine3D==2

== system EKF_MODEL_needfix/Visualization/ISO 15037-1:2006 ==
  VehFdbk : Inport
  Disabled : Subsystem  VariantControl=0
  Enabled : Subsystem  VariantControl=1

== system EKF_MODEL_needfix/model data/Subsystem ==
  In1 : Inport
  In2 : Inport  Port=2
  Gain3 : Gain  Gain=1/18
  model data : Subsystem
  <body_a> : Outport
  <imu> : Outport  Port=2
  <steerangle> : Outport  Port=3
  <EngTrq> : Outport  Port=4
  <xdot> : Outport  Port=5
  <ydot> : Outport  Port=6
  <r> : Outport  Port=7
  wires:
  model data/5(<xdot>) -> <xdot>/1
  model data/2(<body_a>) -> <body_a>/1
  model data/3(<SteerFdbk>) -> Gain3/1
  Gain3/1 -> <steerangle>/1
  In2/1 -> model data/2(In2)
  model data/4(<EngTrq>) -> <EngTrq>/1
  In1/1 -> model data/1(In1)
  model data/6(<ydot>) -> <ydot>/1
  model data/7(<r>) -> <r>/1
  model data/1(<imu>) -> <imu>/1

== system EKF_MODEL_needfix/Controllers/Active Differential Control/No Control ==
  axayaz : Inport
  Steer : Inport  Port=2
  Constant : Constant  Value=0
  Constant1 : Constant  Value=0
  Terminator : Terminator
  Terminator1 : Terminator
  Vector Concatenate2 : Concatenate  NumInputs=4
  DiffPrsCmd : Outport  VectorParamsAs1DForOutWhenUnconnected=off
  TrqCmd : Outport  Port=2  VectorParamsAs1DForOutWhenUnconnected=off
  wires:
  Constant/1 -> Vector Concatenate2/1, Vector Concatenate2/4, Vector Concatenate2/3, Vector Concatenate2/2
  Steer/1 -> Terminator1/1
  Vector Concatenate2/1 -> DiffPrsCmd/1  "DiffPrsCmd"
  axayaz/1 -> Terminator/1
  Constant1/1 -> TrqCmd/1  "TrqCmd"

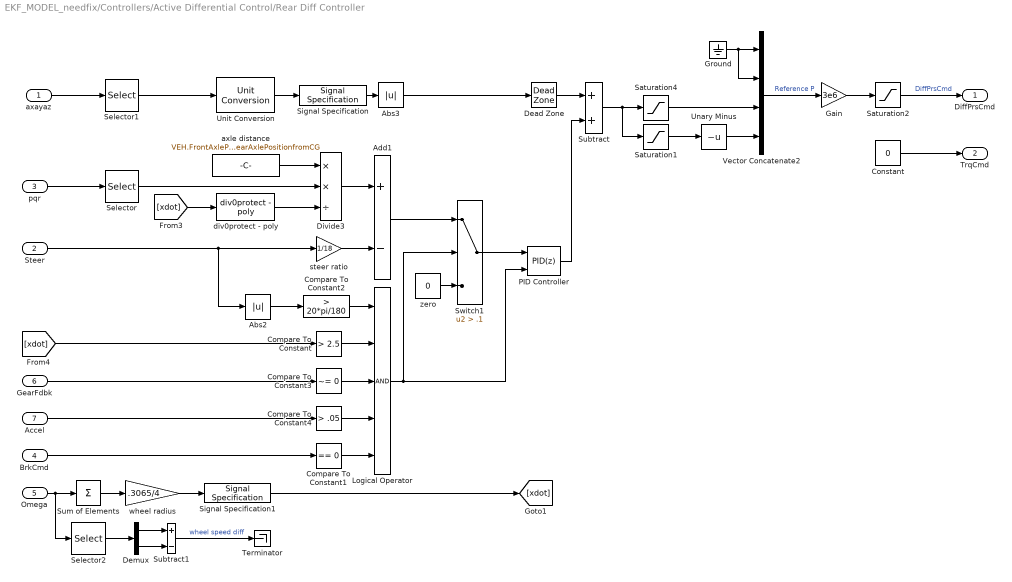
== system EKF_MODEL_needfix/Controllers/Active Differential Control/Rear Diff Controller ==
  axayaz : Inport
  Steer : Inport  Port=2
  pqr : Inport  Port=3
  BrkCmd : Inport  Port=4
  Omega : Inport  Port=5  Unit=rad/s
  GearFdbk : Inport  Port=6
  Accel : Inport  Port=7
  Abs2 : Abs  SaturateOnIntegerOverflow=off
  Abs3 : Abs  ZeroCross=off  SaturateOnIntegerOverflow=off
  Add1 : Sum  Inputs=+-
  Compare To Constant : simulink/Logic and Bit Operations/Compare To Constant  relop=>  const=2.5  OutDataTypeStr=boolean
  Compare To Constant1 : simulink/Logic and Bit Operations/Compare To Constant  relop===  const=0  OutDataTypeStr=boolean
  Compare To Constant2 : simulink/Logic and Bit Operations/Compare To Constant  relop=>  const=20*pi/180  OutDataTypeStr=boolean
  Compare To Constant3 : simulink/Logic and Bit Operations/Compare To Constant  relop=~=  const=0  OutDataTypeStr=boolean
  Compare To Constant4 : simulink/Logic and Bit Operations/Compare To Constant  relop=>  const=.05  OutDataTypeStr=boolean
  Constant : Constant  Value=0
  Dead Zone : DeadZone  ZeroCross=off
  Demux : Demux  Outputs=2
  Divide3 : Product  Inputs=**/
  Gain : Gain  Gain=3e6
  Ground : Ground
  Logical Operator : Logic  Inputs=5  AllPortsSameDT=off  OutDataTypeStr=boolean
  PID Controller : slpidlib/PID Controller  Controller=PID  Form=Parallel  TimeDomain=Discrete-time  UseExternalTs=off  SampleTime=-1  IntegratorMethod=Forward Euler  FilterMethod=Forward Euler  ControllerParametersSource=internal  P=1  I=.05  UseKiTs=off  D=0  N=1  UseFilter=on  TunerSelectOption=Transfer Function Based (PID Tuner App)  ZeroCross=off  InitialConditionSource=internal  InitialConditionForIntegrator=0  InitialConditionForFilter=0  DifferentiatorICPrevScaledInput=0  ExternalReset=either  TrackingMode=off  Kt=1  LimitOutput=on  SatLimitsSource=internal  UpperSaturationLimit=1  LowerSaturationLimit=-1  LinearizeAsGain=on  AntiWindupMode=clamping  Kb=1  LimitIntegrator=off  UpperIntegratorSaturationLimit=inf  LowerIntegratorSaturationLimit=-inf  POutMin=[]  POutMax=[]  IOutMin=[]  IOutMax=[]  DOutMin=[]  DOutMax=[]  NOutMin=[]  NOutMax=[]  SumOutMin=[]  SumOutMax=[]  SaturationOutMin=[]  SaturationOutMax=[]  PParamMin=[]  PParamMax=[]  IParamMin=[]  IParamMax=[]  DParamMin=[]  DParamMax=[]  NParamMin=[]  NParamMax=[]  KbParamMin=[]  KbParamMax=[]  KtParamMin=[]  KtParamMax=[]  KbOutMin=[]  KbOutMax=[]  KtOutMin=[]  KtOutMax=[]  IntegratorOutMin=[]  IntegratorOutMax=[]  FilterOutMin=[]  FilterOutMax=[]  SumI1OutMin=[]  SumI1OutMax=[]  SumI2OutMin=[]  SumI2OutMax=[]  SumI3OutMin=[]  SumI3OutMax=[]  SumI4OutMin=[]  SumI4OutMax=[]  SumDOutMin=[]  SumDOutMax=[]  DifferentiatorOutMin=[]  DifferentiatorOutMax=[]  FilterDiffOutCoefMin=[]  FilterDiffOutCoefMax=[]  ReciprocalOutMin=[]  ReciprocalOutMax=[]  SumDenOutMin=[]  SumDenOutMax=[]  SumNumOutMin=[]  SumNumOutMax=[]  DivideOutMin=[]  DivideOutMax=[]  UdiffTsProdOutMin=[]  UdiffTsProdOutMax=[]  NTsProdOutMin=[]  NTsProdOutMax=[]  UintegralTsProdOutMin=[]  UintegralTsProdOutMax=[]  UngainTsProdOutMin=[]  UngainTsProdOutMax=[]  ClampingZeroOutDataTypeStr=Inherit: Inherit via back propagation  ClampingZeroOutMin=[]  ClampingZeroOutMax=[]  FilterDenConstantOutDataTypeStr=Inherit: Inherit via back propagation  FilterDenConstantOutMin=[]  FilterDenConstantOutMax=[]  PCopyOutDataTypeStr=Inherit: Inherit via back propagation  PCopyOutMin=[]  PCopyOutMax=[]  NCopyOutDataTypeStr=Inherit: Inherit via back propagation  NCopyOutMin=[]  NCopyOutMax=[]  IntegratorContinuousStateAttributes=''  IntegratorStateMustResolveToSignalObject=off  IntegratorRTWStateStorageClass=Auto  FilterContinuousStateAttributes=''  FilterStateMustResolveToSignalObject=off  FilterRTWStateStorageClass=Auto  ParallelPVariant=InternalParameters  IdealPVariant=Disabled  IVariant=InternalParameters  DVariant=InternalParameters  IntegratorVariant=Discrete  SatVariant=Enabled  AWVariant=DiscClampingParallel  PCopyVariant=Disabled  TRVariant=Disabled  FdbkBlocksVariant=Forward  IdealPFdbkVariant=Disabled  SatFdbkVariant=Disabled  DerivativeFilterVariant=ForwardEulerFilter  NVariant=InternalParameters  NCopyVariant=Disabled  FilterICVariant=InternalICsFilter  IntegratorICVariant=InternalICs  ExternalResetVariant=ExternalReset  TRSumVariant=Passthrough  SumFdbkVariant=Disabled  SumVariant=Sum_PID  TsampFilterVariant=InternalTs  TsampNgainVariant=Passthrough  TsampIntegralVariant=Disabled_SignalSpec  ExternalSaturationOutDataTypeStr=Inherit: Same as second input
  Saturation1 : Saturate  UpperLimit=0  LowerLimit=-1  ZeroCross=off
  Saturation2 : Saturate  UpperLimit=5e6  LowerLimit=0  ZeroCross=off
  Saturation4 : Saturate  UpperLimit=1  LowerLimit=0  ZeroCross=off
  Selector : Selector  InputPortWidth=3  IndexOptions=Index vector (dialog)  Indices=[3]  OutputSizes=1
  Selector1 : Selector  InputPortWidth=3  IndexOptions=Index vector (dialog)  Indices=[2]  OutputSizes=1
  Selector2 : Selector  InputPortWidth=4  IndexOptions=Index vector (dialog)  Indices=[3 4]  OutputSizes=1
  Signal Specification : SignalSpecification  Unit=gn
  Signal Specification1 : SignalSpecification  Unit=m/s
  Subtract : Sum
  Subtract1 : Sum  Inputs=+-
  Sum of Elements : Sum  Inputs=+
  Switch1 : Switch  Criteria=u2 > Threshold  Threshold=.1  SaturateOnIntegerOverflow=off  InputSameDT=off
  Terminator : Terminator
  Unary Minus : UnaryMinus
  Unit Conversion : UnitConversion
  Vector Concatenate2 : Concatenate  NumInputs=4
  axle distance : Constant  Value=VEH.FrontAxlePositionfromCG+VEH.RearAxlePositionfromCG
  div0protect - poly : autolibutils/div0protect - poly  thresh=1  ZeroCross1=on  aMode=2
  steer ratio : Gain  Gain=1/18
  wheel radius : Gain  Gain=.3065/4
  zero : Constant  Value=0
  DiffPrsCmd : Outport  VectorParamsAs1DForOutWhenUnconnected=off
  TrqCmd : Outport  Port=2  VectorParamsAs1DForOutWhenUnconnected=off
  wires:
  Vector Concatenate2/1 -> Gain/1  "Reference P"
  Ground/1 -> Vector Concatenate2/2, Vector Concatenate2/1
  Saturation1/1 -> Unary Minus/1
  Gain/1 -> Saturation2/1
  Saturation2/1 -> DiffPrsCmd/1  "DiffPrsCmd"
  Divide3/1 -> Add1/1
  Selector/1 -> Divide3/2
  Logical Operator/1 -> PID Controller/2, Switch1/2
  Switch1/1 -> PID Controller/1
  zero/1 -> Switch1/3
  PID Controller/1 -> Subtract/2
  Add1/1 -> Switch1/1
  axle distance/1 -> Divide3/1
  pqr/1 -> Selector/1
  Compare To Constant2/1 -> Logical Operator/1
  Compare To Constant/1 -> Logical Operator/2
  Abs2/1 -> Compare To Constant2/1
  Steer/1 -> Abs2/1, steer ratio/1
  [xdot] -> Compare To Constant/1
  axayaz/1 -> Selector1/1
  Sum of Elements/1 -> wheel radius/1
  wheel radius/1 -> Signal Specification1/1
  Omega/1 -> Selector2/1, Sum of Elements/1
  Signal Specification1/1 -> [xdot]
  BrkCmd/1 -> Compare To Constant1/1
  GearFdbk/1 -> Compare To Constant3/1
  Compare To Constant3/1 -> Logical Operator/3
  Subtract/1 -> Saturation1/1, Saturation4/1
  Accel/1 -> Compare To Constant4/1
  Compare To Constant4/1 -> Logical Operator/4
  steer ratio/1 -> Add1/2
  Saturation4/1 -> Vector Concatenate2/3
  Selector1/1 -> Unit Conversion/1
  Signal Specification/1 -> Abs3/1
  Abs3/1 -> Dead Zone/1
  Dead Zone/1 -> Subtract/1
  Constant/1 -> TrqCmd/1
  Selector2/1 -> Demux/1
  Demux/1 -> Subtract1/1
  Demux/2 -> Subtract1/2
  Unary Minus/1 -> Vector Concatenate2/4
  Subtract1/1 -> Terminator/1  "wheel speed diff"
  Compare To Constant1/1 -> Logical Operator/5
  Unit Conversion/1 -> Signal Specification/1
  [xdot] -> div0protect - poly/1
  div0protect - poly/1 -> Divide3/3

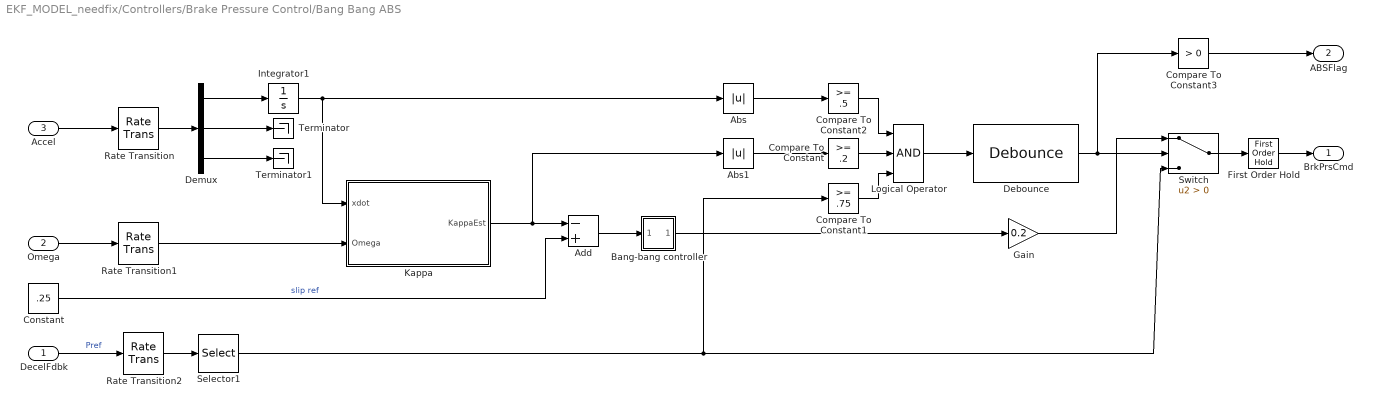
== system EKF_MODEL_needfix/Controllers/Brake Pressure Control/Bang Bang ABS ==
  DecelFdbk : Inport
  Omega : Inport  Port=2
  Accel : Inport  Port=3
  Abs : Abs  SaturateOnIntegerOverflow=off
  Abs1 : Abs  SaturateOnIntegerOverflow=off
  Add : Sum  Inputs=-+
  Bang-bang controller : Subsystem  mask(Sign){}
      mask help: y = sign(x)
      mask Help: Sign Function:\n\t\t\ty = 1 if x > 0\n\t\t\ty = 0 if x = 0\n\t\t\ty = -1 if x < 0
      mask Display: plot(-50,-50,50,50,[-50,50],[0,0],[0,0],[-50,50],[-40,0],[-30,-30],[0,40],[30,30])
  Compare To Constant : simulink/Logic and Bit Operations/Compare To Constant  relop=>=  const=.2  OutDataTypeStr=boolean
  Compare To Constant1 : simulink/Logic and Bit Operations/Compare To Constant  relop=>=  const=.75  OutDataTypeStr=boolean
  Compare To Constant2 : simulink/Logic and Bit Operations/Compare To Constant  relop=>=  const=.5  OutDataTypeStr=boolean
  Compare To Constant3 : simulink/Logic and Bit Operations/Compare To Constant  relop=>  const=0  OutDataTypeStr=boolean  ZeroCross=off
  Constant : Constant  Value=.25
  Debounce : autolibutils/Debounce  DbcOn_Cnts=.1*.001  DbcOff_Cnts=.1*.001  aMode=2
  Demux : Demux  Outputs=3
  First Order Hold : FirstOrderHold  ErrorTolerance=1
  Gain : Gain  Gain=0.2
  Integrator1 : Integrator
  Kappa : Subsystem  TreatAsAtomicUnit=on
  Logical Operator : Logic  Inputs=3  AllPortsSameDT=off  OutDataTypeStr=boolean
  Rate Transition : RateTransition  Deterministic=off  OutPortSampleTime=.001
  Rate Transition1 : RateTransition  Deterministic=off  OutPortSampleTime=.001
  Rate Transition2 : RateTransition  Deterministic=off  OutPortSampleTime=.001
  Selector1 : Selector  InputPortWidth=1  IndexOptions=Index vector (dialog)  Indices=[1 1 1 1]  OutputSizes=1
  Switch : Switch  Criteria=u2 > Threshold  ZeroCross=off  SaturateOnIntegerOverflow=off  InputSameDT=off
  Terminator : Terminator
  Terminator1 : Terminator
  BrkPrsCmd : Outport  VectorParamsAs1DForOutWhenUnconnected=off
  ABSFlag : Outport  Port=2
  wires:
  Bang-bang controller/1(out_1) -> Gain/1
  Add/1 -> Bang-bang controller/1(in_1)
  First Order Hold/1 -> BrkPrsCmd/1
  DecelFdbk/1 -> Rate Transition2/1  "Pref"
  Constant/1 -> Add/2  "slip ref"
  Switch/1 -> First Order Hold/1
  Kappa/1(KappaEst) -> Add/1, Abs1/1
  Logical Operator/1 -> Debounce/1
  Compare To Constant/1 -> Logical Operator/2
  Compare To Constant1/1 -> Logical Operator/3
  Debounce/1 -> Compare To Constant3/1, Switch/2
  Abs/1 -> Compare To Constant2/1
  Compare To Constant2/1 -> Logical Operator/1
  Gain/1 -> Switch/1
  Integrator1/1 -> Kappa/1(xdot), Abs/1
  Demux/2 -> Terminator/1
  Accel/1 -> Rate Transition/1
  Demux/1 -> Integrator1/1
  Rate Transition/1 -> Demux/1
  Demux/3 -> Terminator1/1
  Omega/1 -> Rate Transition1/1
  Rate Transition1/1 -> Kappa/2(Omega)
  Rate Transition2/1 -> Selector1/1
  Compare To Constant3/1 -> ABSFlag/1
  Selector1/1 -> Compare To Constant1/1, Switch/3
  Abs1/1 -> Compare To Constant/1
